simulink model "AHRS_Type4_d01_Pordal"  (R2022b)
settings: Solver=FixedStepDiscrete  StartTime=0.0  StopTime=ft  FixedStep=st  RelTol=1e-3
InitFcn:
  | load("AHRSDataset_2.mat");
  | IMU = IMU_true;
  | Magnetometer = MAG_true(:,2:4);
  | Euler_true = NavData(2:end,end-2:end)*pi/180;
  | % Parameters
  | g = 9.7803; % m/s^2
  | st = 0.01; % (s) Sample Time
  | ft = size(IMU_true,1)*st-st; % Final Time
  | time = 0:st:ft; % Simulation Time
  | a_acc__B = [time' IMU(:,2:4)];
  | om_gyro__B = [time' IMU(:,5:7)];
  | m_mag__B = [time' Magnetometer];
  | Euler_true = [time' Euler_true];
libraries: simulink_extras x3, matrix_library x1, simulink x1
settings Model: Creator=reza  LastModifiedBy=reza
settings DataIOCC: ReturnWorkspaceOutputs=off

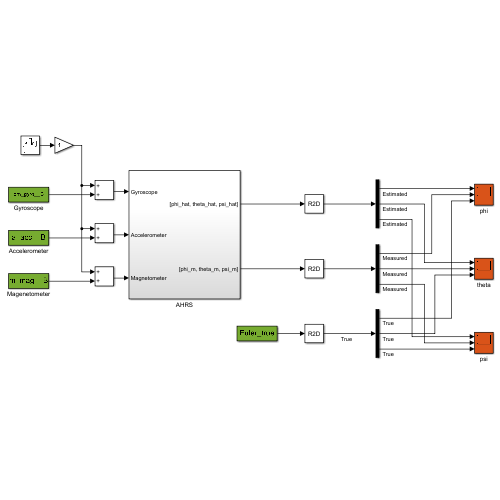
[thumbnail: Simulink's stored preview of the top-level diagram]
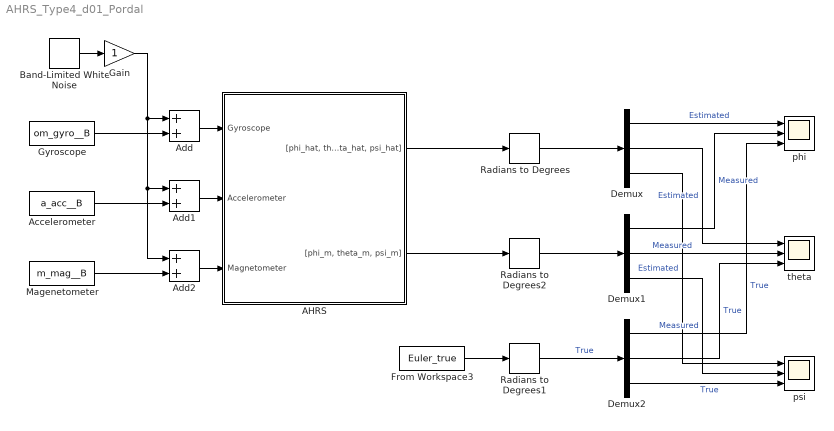
== system AHRS_Type4_d01_Pordal ==
  AHRS : Subsystem
  Accelerometer : FromWorkspace  VariableName=a_acc__B  SampleTime=st
  Add : Sum
  Add1 : Sum
  Add2 : Sum
  Band-Limited White Noise : simulink/Sources/Band-Limited White Noise  Cov=1e-5  Ts=0.01  seed=[23341]
  Demux : Demux  Outputs=3
  Demux1 : Demux  Outputs=3
  Demux2 : Demux  Outputs=3
  From Workspace3 : FromWorkspace  VariableName=Euler_true  SampleTime=st
  Gain : Gain
  Gyroscope : FromWorkspace  VariableName=om_gyro__B  SampleTime=st
  Magenetometer : FromWorkspace  VariableName=m_mag__B  SampleTime=st
  Radians to Degrees : simulink_extras/Transformations/Radians to Degrees
  Radians to Degrees1 : simulink_extras/Transformations/Radians to Degrees
  Radians to Degrees2 : simulink_extras/Transformations/Radians to Degrees
  phi : Scope  NumInputPorts=3
  psi : Scope  NumInputPorts=3
  theta : Scope  NumInputPorts=3
  wires:
  Magenetometer/1 -> Add2/2
  Radians to Degrees/1 -> Demux/1
  AHRS/1("[phi_hat, theta_hat, psi_hat]") -> Radians to Degrees/1
  Add/1 -> AHRS/1(Gyroscope)
  Band-Limited White Noise/1 -> Gain/1
  Gyroscope/1 -> Add/2
  Add1/1 -> AHRS/2(Accelerometer)
  Accelerometer/1 -> Add1/2
  Gain/1 -> Add1/1, Add2/1, Add/1
  From Workspace3/1 -> Radians to Degrees1/1
  Radians to Degrees1/1 -> Demux2/1  "True"
  Add2/1 -> AHRS/3(Magnetometer)
  AHRS/2("[phi_m, theta_m, psi_m]") -> Radians to Degrees2/1
  Radians to Degrees2/1 -> Demux1/1
  Demux/1 -> phi/1  "Estimated"
  Demux1/1 -> phi/2  "Measured"
  Demux2/1 -> phi/3  "True"
  Demux/2 -> theta/1  "Estimated"
  Demux1/2 -> theta/2  "Measured"
  Demux2/2 -> theta/3  "True"
  Demux2/3 -> psi/3  "True"
  Demux/3 -> psi/1  "Estimated"
  Demux1/3 -> psi/2  "Measured"

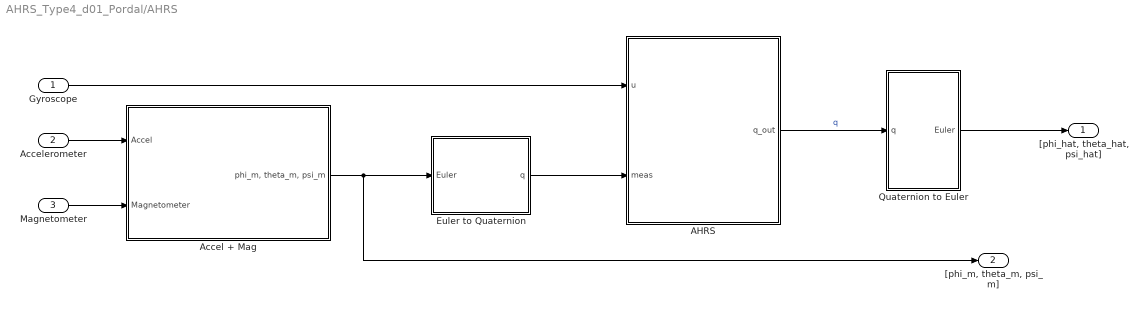
== system AHRS_Type4_d01_Pordal/AHRS ==
  Gyroscope : Inport
  Accelerometer : Inport  Port=2
  Magnetometer : Inport  Port=3
  AHRS : MATLAB Function  TreatAsAtomicUnit=on
  Accel + Mag : Subsystem
  Euler to Quaternion : MATLAB Function  TreatAsAtomicUnit=on
  Quaternion to Euler : MATLAB Function  TreatAsAtomicUnit=on
  "[phi_hat, theta_hat, psi_hat]" : Outport
  "[phi_m, theta_m, psi_m]" : Outport  Port=2
  wires:
  AHRS/1(q_out) -> Quaternion to Euler/1(q)  "q"
  Accelerometer/1 -> Accel + Mag/1(Accel)
  Magnetometer/1 -> Accel + Mag/2(Magnetometer)
  Gyroscope/1 -> AHRS/1(u)
  Accel + Mag/1("phi_m, theta_m, psi_m") -> "[phi_m, theta_m, psi_m]"/1, Euler to Quaternion/1(Euler)
  Quaternion to Euler/1(Euler) -> "[phi_hat, theta_hat, psi_hat]"/1
  Euler to Quaternion/1(q) -> AHRS/2(meas)

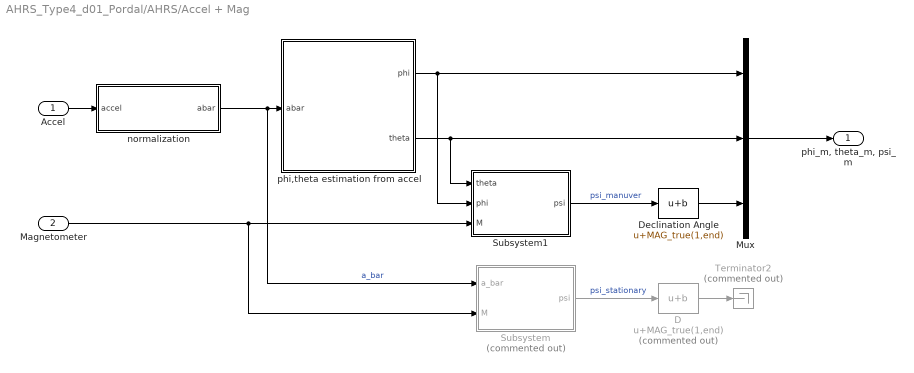
== system AHRS_Type4_d01_Pordal/AHRS/Accel + Mag ==
  Accel : Inport
  Magnetometer : Inport  Port=2
  D : Bias  Commented=on  Bias=MAG_true(1,end)  SaturateOnIntegerOverflow=off
  Declination Angle : Bias  Bias=MAG_true(1,end)  SaturateOnIntegerOverflow=off
  Mux : Mux  Inputs=3
  Subsystem : Subsystem  Commented=on
  Subsystem1 : Subsystem
  Terminator2 : Terminator  Commented=on
  normalization : Subsystem
  phi,theta estimation from accel : Subsystem
  "phi_m, theta_m, psi_m" : Outport
  wires:
  phi,theta estimation from accel/2(theta) -> Mux/2, Subsystem1/1(theta)
  Mux/1 -> "phi_m, theta_m, psi_m"/1
  normalization/1(abar) -> Subsystem/1(a_bar), phi,theta estimation from accel/1(abar)  "a_bar"
  Accel/1 -> normalization/1(accel)
  Magnetometer/1 -> Subsystem/2(M), Subsystem1/3(M)
  Subsystem/1(psi) -> D/1  "psi_stationary"
  phi,theta estimation from accel/1(phi) -> Mux/1, Subsystem1/2(phi)
  Subsystem1/1(psi) -> Declination Angle/1  "psi_manuver"
  Declination Angle/1 -> Mux/3
  D/1 -> Terminator2/1

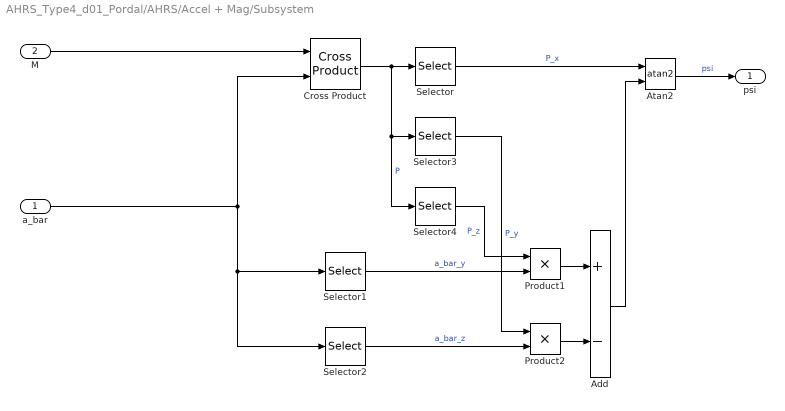
== system AHRS_Type4_d01_Pordal/AHRS/Accel + Mag/Subsystem ==
  a_bar : Inport
  M : Inport  Port=2
  Add : Sum  Inputs=+-
  Atan2 : Trigonometry  Operator=atan2
  Cross Product : matrix_library/Cross Product
  Product1 : Product
  Product2 : Product
  Selector : Selector  InputPortWidth=3  IndexOptions=Index vector (dialog)  Indices=1  OutputSizes=1
  Selector1 : Selector  InputPortWidth=3  IndexOptions=Index vector (dialog)  Indices=2  OutputSizes=1
  Selector2 : Selector  InputPortWidth=3  IndexOptions=Index vector (dialog)  Indices=3  OutputSizes=1
  Selector3 : Selector  InputPortWidth=3  IndexOptions=Index vector (dialog)  Indices=2  OutputSizes=1
  Selector4 : Selector  InputPortWidth=3  IndexOptions=Index vector (dialog)  Indices=3  OutputSizes=1
  psi : Outport
  wires:
  Selector1/1 -> Product1/2  "a_bar_y"
  Selector2/1 -> Product2/2  "a_bar_z"
  Cross Product/1 -> Selector3/1, Selector4/1, Selector/1  "P"
  Product2/1 -> Add/2
  a_bar/1 -> Cross Product/2, Selector2/1, Selector1/1
  Selector4/1 -> Product1/1  "P_z"
  Product1/1 -> Add/1
  Selector/1 -> Atan2/1  "P_x"
  Add/1 -> Atan2/2
  Selector3/1 -> Product2/1  "P_y"
  Atan2/1 -> psi/1  "psi"
  M/1 -> Cross Product/1

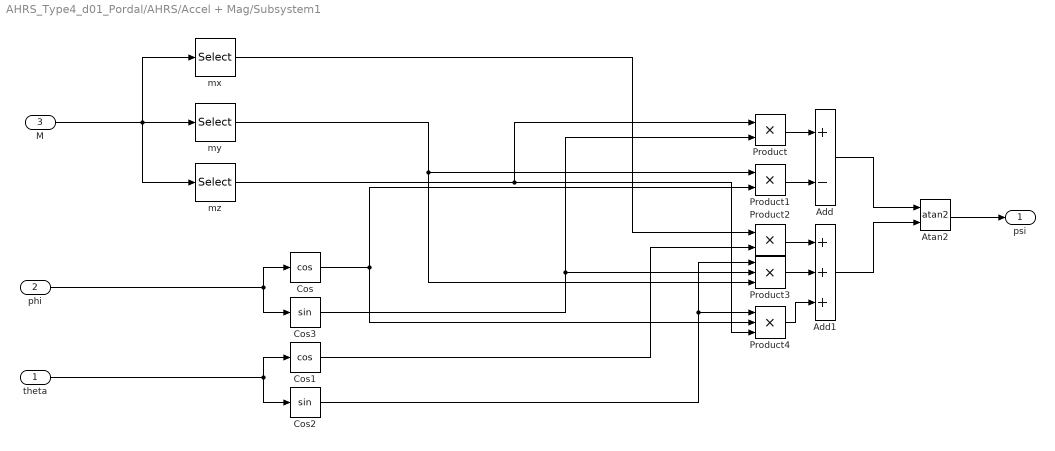
== system AHRS_Type4_d01_Pordal/AHRS/Accel + Mag/Subsystem1 ==
  theta : Inport
  phi : Inport  Port=2
  M : Inport  Port=3
  Add : Sum  Inputs=+-
  Add1 : Sum  Inputs=+++
  Atan2 : Trigonometry  Operator=atan2
  Cos : Trigonometry  Operator=cos
  Cos1 : Trigonometry  Operator=cos
  Cos2 : Trigonometry
  Cos3 : Trigonometry
  Product : Product
  Product1 : Product
  Product2 : Product
  Product3 : Product  Inputs=3
  Product4 : Product  Inputs=3
  mx : Selector  InputPortWidth=3  IndexOptions=Index vector (dialog)  Indices=1  OutputSizes=1
  my : Selector  InputPortWidth=3  IndexOptions=Index vector (dialog)  Indices=2  OutputSizes=1
  mz : Selector  InputPortWidth=3  IndexOptions=Index vector (dialog)  Indices=3  OutputSizes=1
  psi : Outport
  wires:
  phi/1 -> Cos3/1, Cos/1
  theta/1 -> Cos1/1, Cos2/1
  M/1 -> my/1, mz/1, mx/1
  Add/1 -> Atan2/1
  Add1/1 -> Atan2/2
  Product/1 -> Add/1
  Cos3/1 -> Product3/2, Product/2
  mz/1 -> Product/1, Product4/3
  Product1/1 -> Add/2
  Cos/1 -> Product4/2, Product1/2
  my/1 -> Product1/1, Product3/3
  Cos1/1 -> Product2/2
  Product2/1 -> Add1/1
  Product3/1 -> Add1/2
  Product4/1 -> Add1/3
  mx/1 -> Product2/1
  Cos2/1 -> Product3/1, Product4/1
  Atan2/1 -> psi/1

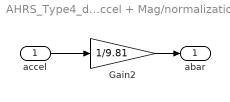
== system AHRS_Type4_d01_Pordal/AHRS/Accel + Mag/normalization ==
  accel : Inport
  Gain2 : Gain  Gain=1/9.81
  abar : Outport
  wires:
  Gain2/1 -> abar/1
  accel/1 -> Gain2/1

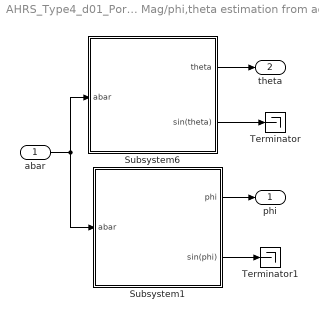
== system AHRS_Type4_d01_Pordal/AHRS/Accel + Mag/phi,theta estimation from accel ==
  abar : Inport
  Subsystem1 : Subsystem
  Subsystem6 : Subsystem
  Terminator : Terminator
  Terminator1 : Terminator
  phi : Outport
  theta : Outport  Port=2
  wires:
  Subsystem1/1(phi) -> phi/1
  Subsystem6/1(theta) -> theta/1
  abar/1 -> Subsystem6/1(abar), Subsystem1/1(abar)
  Subsystem1/2(sin(phi)) -> Terminator1/1
  Subsystem6/2(sin(theta)) -> Terminator/1

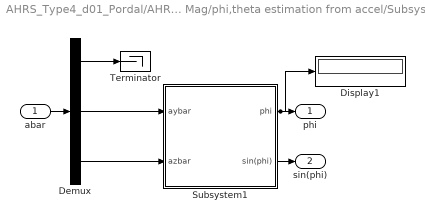
== system AHRS_Type4_d01_Pordal/AHRS/Accel + Mag/phi,theta estimation from accel/Subsystem1 ==
  abar : Inport
  Demux : Demux  Outputs=3
  Display1 : Display
  Subsystem1 : Subsystem
  Terminator : Terminator
  phi : Outport
  sin(phi) : Outport  Port=2
  wires:
  Subsystem1/1(phi) -> phi/1, Display1/1
  Subsystem1/2(sin(phi)) -> sin(phi)/1
  Demux/3 -> Subsystem1/2(azbar)
  Demux/2 -> Subsystem1/1(aybar)
  abar/1 -> Demux/1
  Demux/1 -> Terminator/1

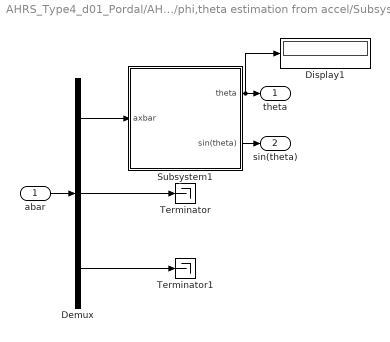
== system AHRS_Type4_d01_Pordal/AHRS/Accel + Mag/phi,theta estimation from accel/Subsystem6 ==
  abar : Inport
  Demux : Demux  Outputs=3
  Display1 : Display
  Subsystem1 : Subsystem
  Terminator : Terminator
  Terminator1 : Terminator
  theta : Outport
  sin(theta) : Outport  Port=2
  wires:
  Demux/3 -> Terminator1/1
  Demux/2 -> Terminator/1
  abar/1 -> Demux/1
  Subsystem1/2(sin(theta)) -> sin(theta)/1
  Subsystem1/1(theta) -> theta/1, Display1/1
  Demux/1 -> Subsystem1/1(axbar)

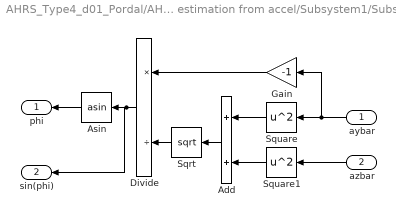
== system AHRS_Type4_d01_Pordal/AHRS/Accel + Mag/phi,theta estimation from accel/Subsystem1/Subsystem1 ==
  aybar : Inport
  azbar : Inport  Port=2
  Add : Sum
  Asin : Trigonometry  Operator=asin
  Divide : Product  Inputs=*/
  Gain : Gain  Gain=-1
  Sqrt : Sqrt
  Square : Math  Operator=square
  Square1 : Math  Operator=square
  phi : Outport
  sin(phi) : Outport  Port=2
  wires:
  Divide/1 -> Asin/1, sin(phi)/1
  Gain/1 -> Divide/1
  Sqrt/1 -> Divide/2
  Add/1 -> Sqrt/1
  Square1/1 -> Add/2
  Square/1 -> Add/1
  azbar/1 -> Square1/1
  aybar/1 -> Square/1, Gain/1
  Asin/1 -> phi/1

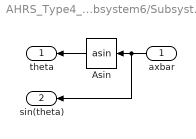
== system AHRS_Type4_d01_Pordal/AHRS/Accel + Mag/phi,theta estimation from accel/Subsystem6/Subsystem1 ==
  axbar : Inport
  Asin : Trigonometry  Operator=asin
  theta : Outport
  sin(theta) : Outport  Port=2
  wires:
  Asin/1 -> theta/1
  axbar/1 -> Asin/1, sin(theta)/1

== matlab function AHRS_Type4_d01_Pordal/AHRS/Euler to Quaternion ==
  data: Euler input; q output
function q = fcn(Euler)

phi = Euler(1);
theta = Euler(2);
psi = Euler(3);

q0 = cos(psi/2)*cos(theta/2)*cos(phi/2) + sin(psi/2)*sin(theta/2)*sin(phi/2);
q1 = cos(psi/2)*cos(theta/2)*sin(phi/2) - sin(psi/2)*sin(theta/2)*cos(phi/2);
q2 = cos(psi/2)*sin(theta/2)*cos(phi/2) + sin(psi/2)*cos(theta/2)*sin(phi/2);
q3 = sin(psi/2)*cos(theta/2)*cos(phi/2) - cos(psi/2)*sin(theta/2)*sin(phi/2);

q = [q0, q1, q2, q3];

end

== matlab function AHRS_Type4_d01_Pordal/AHRS/Quaternion to Euler ==
  data: q input; Euler output
function Euler = fcn(q)

q0 = q(1);
q1 = q(2);
q2 = q(3);
q3 = q(4);

phi = atan2(2*(q0*q1 + q2*q3), (q0^2 + q3^2 - q1^2 - q2^2));
theta = asin(2*(q0*q2 - q1*q3));
psi = atan2(2*(q0*q3 + q1*q2), (q0^2 + q1^2 - q2^2 - q3^2));

Euler = [phi, theta, psi];

end

== matlab function AHRS_Type4_d01_Pordal/AHRS/AHRS ==
  settings: updateMethod=DISCRETE
  data: u input; meas input; q_out output
function q_out = fcn(u, meas)

q0 = meas(1);
q1 = meas(2);
q2 = meas(3);
q3 = meas(4);

p = u(1);
q = u(2);
r = u(3);

y_m = [q0; q1; q2; q3];

Ts = 0.01;
    
    Q = 1e-4*[1 0 0 0
              0 1 0 0
              0 0 1 0
              0 0 0 1];

    R = 1e-1*[1 0 0 0
              0 1 0 0
              0 0 1 0
              0 0 0 1];

    persistent q_hat P
    
    if isempty(q_hat)
        q_hat = [q0; q1; q2; q3];
    end

    if isempty(P)
        P=[ 10 0 0 0
            0 10 0 0
            0 0 10 0
            0 0 0 10];
    end

%%
    q_hat = q_hat + 0.5*Ts*[0 -p -q -r; p 0 r -q; q -r 0 p; r q -p 0]*q_hat;
    %%
    A = 0.5*Ts*[0 -p -q -r; p 0 r -q; q -r 0 p; r q -p 0];
    F = eye(4) + A;
    P = F*P*F'+ Q;
    %%

    y_hat = q_hat;
    C = eye(4);
    K = P*C'*inv(C*P*C' + R);
    q_hat = q_hat + K*(y_m - y_hat);
    P = (eye(4) - K*C)*P*(eye(4) - K*C)' + K*R*K';

    q_out = q_hat;
end
